simulink model "SD_RX"  (R2020a)
settings: Solver=VariableStepAuto  StartTime=0.0  StopTime=500  RelTol=1e-3
undefined symbols (not defined in the file): doppler
libraries: commchan3 x2, commdigbbndpm3 x2, commrandsrc3 x1, commsink2 x1
settings Model: Creator=ja545  LastModifiedBy=jose_
settings SFSimCC: CustomCodeUndefinedFunction=UseInterfaceOnly

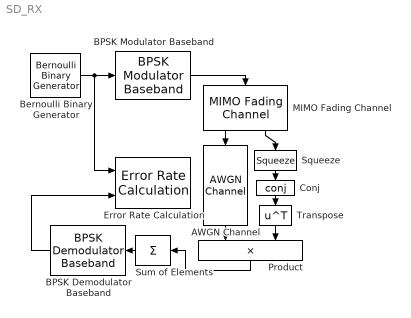
== system SD_RX ==
  AWGN Channel : commchan3/AWGN Channel  InputProcessing=Columns as channels (frame based)  seed=67  noiseMode="Signal to noise ratio  (Eb/No)"  EbNodB=EbNo  EsNodB=10  SNRdB=10  bitsPerSym=1  Ps=1  Tsym=0.01  variance=1
  BPSK Demodulator Baseband : commdigbbndpm3/BPSK Demodulator Baseband  DecType=Hard decision  VarSource=Dialog  Variance=1  Ph=0  outDtype=Inherit via internal rule  derotateFactorWordLen=16  derotateFactorDataTypeStr=Inherit: Same word length as input  derotateFactorLastDataTypeStr=Inherit: Same word length as input
  BPSK Modulator Baseband : commdigbbndpm3/BPSK Modulator Baseband  Ph=0  outDtype=double  outWordLen=16  outUDDataType=sfix(16)  outFracLenMode=Best precision  outFracLen=15  outDataTypeStr=double  outLastDataTypeStr=double
  Bernoulli Binary Generator : commrandsrc3/Bernoulli Binary Generator  ProbabilityOfZero=0.5  SeedSource=Auto  Seed=0  SampleTime=0.01  SamplesPerFrame=1  OutputDataType=double  SimulateUsing=Interpreted execution
  Conj : Math  Operator=conj  SignedPower=on  SaturateOnIntegerOverflow=on
  Error Rate Calculation : commsink2/Error Rate Calculation  N=0  st_delay=0  cp_mode=Entire frame  subframe=[]  PMode=Workspace  WsName=ErrorVec  RsMode2=off  stop=off  numErr=100  maxBits=1e6
  MIMO Fading Channel : commchan3/MIMO Fading Channel  InheritSampleRate=on  SampleRate=1  PathDelays=0.00001  AveragePathGains=0  NormalizePathGains=on  FadingDistribution=Rayleigh  KFactor=3  DirectPathDopplerShift=0  DirectPathInitialPhase=0  MaximumDopplerShift=5  DopplerSpectrum=doppler('Jakes')  SpatialCorrelationSpecification=None  SpatialCorrelationMatrix=[1 0 0 0; 0 1 0 0; 0 0 1 0; 0 0 0 1]  NumTransmitAntennas=1  NumReceiveAntennas=4  TransmitCorrelationMatrix=[1 0; 0 1]  ReceiveCorrelationMatrix=[1 0; 0 1]  AntennaSelection=Off  NormalizeChannelOutputs=off  SimulateUsing=Interpreted execution  FadingTechnique=Filtered Gaussian noise  NumSinusoids=48  InitialTimeSource=Property  InitialTime=0  RandomStream=mt19937ar with seed  Seed=73  PathGainsOutputPort=on  Visualization=Off  AntennaPairsToDisplay=[ 1, 1 ]  PathsForDopplerDisplay=1  SamplesToDisplay=25%
      settings: SourceProductBaseCode=CM
  Product : Product
  Squeeze : Squeeze
  Sum of Elements : Sum  Inputs=+
  Transpose : Math  Operator=transpose  SignedPower=on  SaturateOnIntegerOverflow=on
  wires:
  Bernoulli Binary Generator/1 -> Error Rate Calculation/1, BPSK Modulator Baseband/1
  MIMO Fading Channel/1 -> AWGN Channel/1
  BPSK Demodulator Baseband/1 -> Error Rate Calculation/2
  Sum of Elements/1 -> BPSK Demodulator Baseband/1
  Product/1 -> Sum of Elements/1
  Conj/1 -> Transpose/1
  Squeeze/1 -> Conj/1
  MIMO Fading Channel/2 -> Squeeze/1
  BPSK Modulator Baseband/1 -> MIMO Fading Channel/1
  Transpose/1 -> Product/2
  AWGN Channel/1 -> Product/1
